simulink model "Fault_Analyzer_Example_FaultModel"  (R2025b)
settings: Solver=VariableStepAuto  StartTime=0.0  StopTime=10.0  RelTol=1e-3  EnableMultiTasking=on
settings Model: Creator=P28500  LastModifiedBy=P28500
settings DebuggingCC: InheritedTsInSrcMsg=none

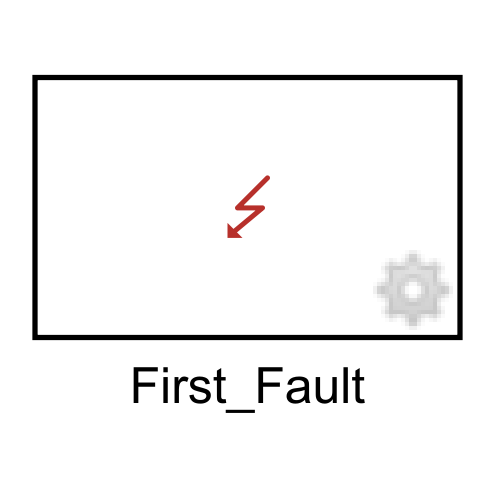
[thumbnail: Simulink's stored preview of the top-level diagram]
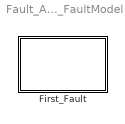
== system Fault_Analyzer_Example_FaultModel ==
  First_Fault : Subsystem  TreatAsAtomicUnit=on  IsInjectorSS=on

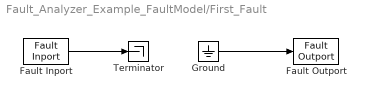
== system Fault_Analyzer_Example_FaultModel/First_Fault ==
  Fault Inport : FaultInport
  Fault Outport : FaultOutport
  Ground : Ground
  Terminator : Terminator
  wires:
  Ground/1 -> Fault Outport/1
  Fault Inport/1 -> Terminator/1
